simulink model "testgood"  (R2017b)
settings: Solver=VariableStepAuto  StartTime=0.0  StopTime=inf  RelTol=1e-3
libraries: dspnetwork x1, etargetslib x1
settings Model: Creator=E6320  LastModifiedBy=E6320
settings DataIOCC: SaveOutput=off  SignalLogging=off  DSMLogging=off  SaveTime=off
settings CodeAppCC: StateflowObjectComments=on

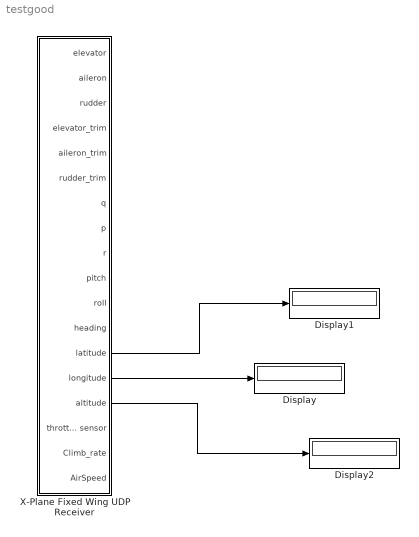
== system testgood ==
  Display : Display
  Display1 : Display
  Display2 : Display
  X-Plane Fixed Wing UDP Receiver : Subsystem  AncestorBlock=X_Plane_Communication_Library/Fixed Wing/X-Plane Fixed Wing UDP Receiver  mask{ip_adress='127.0.0.1', port_number=49004}
      mask prompts: ip_adress "Local IP Adress (default: '127.0.0.1' )"; port_number "Output Port Number (defaut: '49004')"
      mask help: This block is configured to receiver data from a fixed wing aircraft on X-Plane Flight Simulator.
      mask Help: Contact adrianobittar@gmail.com
  wires:
  X-Plane Fixed Wing UDP Receiver/14(longitude) -> Display/1
  X-Plane Fixed Wing UDP Receiver/13(latitude) -> Display1/1
  X-Plane Fixed Wing UDP Receiver/15(altitude) -> Display2/1

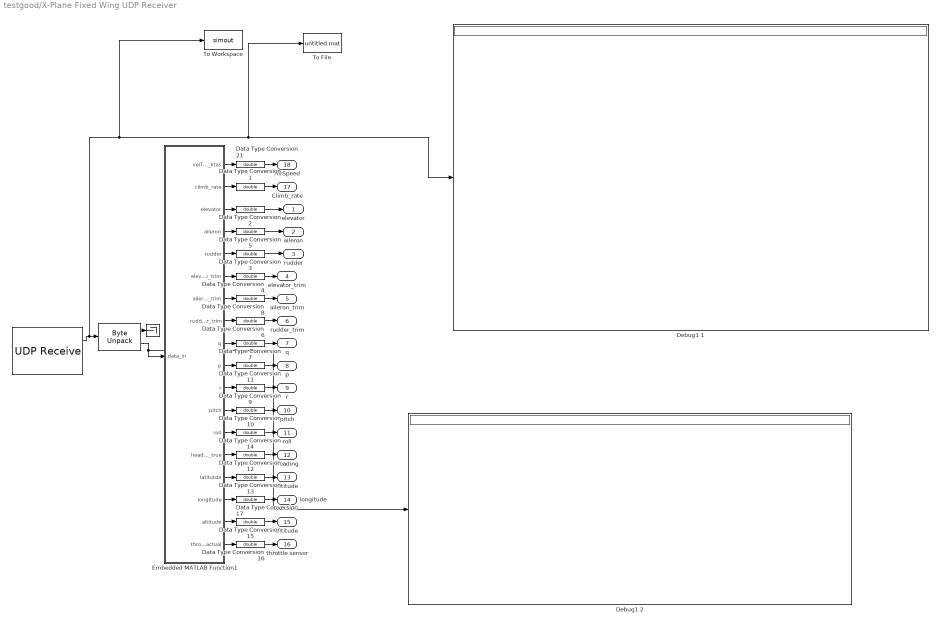
== system testgood/X-Plane Fixed Wing UDP Receiver ==
  " " : Terminator
  "    " : dspnetwork/UDP Receive  localURL='0.0.0.0'  localPort=port_number  remoteURL=ip_adress  remotePort=-1  recvBufferSize=8192  dims=293  signalDatatype=uint8  isVarSize=off  showBlockingTime=on  blockingTime=20  sampletime=0.02  blockPlatform=WINDOWS
      settings: SourceProductName=DSP System Toolbox  SourceProductBaseCode=DS
  "     " : etargetslib/Byte Unpack  dimensions={5,[9,8]}  datatypes={'uint8','single'}  byteAlign=1
  Data Type Conversion{1..17,21} (18 alike) : DataTypeConversion  OutDataTypeStr=double  SaturateOnIntegerOverflow=on
  Debug1 1 : Display
  Debug1 2 : Display
  Embedded MATLAB Function1 : MATLAB Function  TreatAsAtomicUnit=on
  To File : ToFile  SaveFormat=Timeseries
  To Workspace : ToWorkspace  VariableName=simout  SaveFormat=Timeseries  SampleTime=-1
  "elevator " : Outport
  aileron : Outport  Port=2
  rudder : Outport  Port=3
  elevator_trim : Outport  Port=4
  aileron_trim : Outport  Port=5
  rudder_trim : Outport  Port=6
  q : Outport  Port=7
  p : Outport  Port=8
  r : Outport  Port=9
  pitch : Outport  Port=10
  roll : Outport  Port=11
  heading : Outport  Port=12
  latitude : Outport  Port=13
  longitude : Outport  Port=14
  altitude : Outport  Port=15
  throttle sensor : Outport  Port=16
  Climb_rate : Outport  Port=17
  AirSpeed : Outport  Port=18
  wires:
  Data Type Conversion11/1 -> p/1
  Data Type Conversion16/1 -> throttle sensor/1
  Data Type Conversion15/1 -> altitude/1
  Data Type Conversion17/1 -> longitude/1
  Data Type Conversion14/1 -> roll/1
  Data Type Conversion13/1 -> latitude/1
  Data Type Conversion12/1 -> heading/1
  Data Type Conversion7/1 -> q/1
  Data Type Conversion6/1 -> rudder_trim/1
  Data Type Conversion4/1 -> elevator_trim/1
  Data Type Conversion3/1 -> rudder/1
  Data Type Conversion8/1 -> aileron_trim/1
  Data Type Conversion5/1 -> aileron/1
  Data Type Conversion2/1 -> "elevator "/1
  Data Type Conversion1/1 -> Climb_rate/1
  Data Type Conversion21/1 -> AirSpeed/1
  Embedded MATLAB Function1/2(climb_rate) -> Data Type Conversion1/1
  Embedded MATLAB Function1/3(elevator) -> Data Type Conversion2/1
  Embedded MATLAB Function1/4(aileron) -> Data Type Conversion5/1
  Embedded MATLAB Function1/5(rudder) -> Data Type Conversion3/1
  Embedded MATLAB Function1/6(elevator_trim) -> Data Type Conversion4/1
  Embedded MATLAB Function1/7(aileron_trim) -> Data Type Conversion8/1
  Embedded MATLAB Function1/8(rudder_trim) -> Data Type Conversion6/1
  Embedded MATLAB Function1/9(q) -> Data Type Conversion7/1
  Embedded MATLAB Function1/10(p) -> Data Type Conversion11/1
  Embedded MATLAB Function1/11(r) -> Data Type Conversion9/1
  Embedded MATLAB Function1/12(pitch) -> Data Type Conversion10/1
  Embedded MATLAB Function1/13(roll) -> Data Type Conversion14/1
  Embedded MATLAB Function1/14(heading_true) -> Data Type Conversion12/1
  Embedded MATLAB Function1/15(latitutde) -> Data Type Conversion13/1
  Embedded MATLAB Function1/16(longitude) -> Data Type Conversion17/1
  Embedded MATLAB Function1/17(altitude) -> Data Type Conversion15/1
  Embedded MATLAB Function1/18(throttle_actual) -> Data Type Conversion16/1
  Embedded MATLAB Function1/1(velTrue_ktas) -> Data Type Conversion21/1
  "     "/1 -> " "/1
  Data Type Conversion10/1 -> pitch/1
  "    "/1 -> To Workspace/1, To File/1, Debug1 1/1, "     "/1
  Data Type Conversion9/1 -> r/1
  "     "/2 -> Debug1 2/1, Embedded MATLAB Function1/1(data_in)

== matlab function testgood/X-Plane Fixed Wing UDP Receiver/Embedded MATLAB Function1 ==
  data: velTrue_ktas output; climb_rate output; data_in input; elevator output; aileron output; rudder output; elevator_trim output; aileron_trim output; rudder_trim output; q output; p output; r output; pitch output; roll output; heading_true output; latitutde output; longitude output; altitude output; throttle_actual output
function [velTrue_ktas, climb_rate,elevator, aileron, rudder, elevator_trim, aileron_trim, rudder_trim, q,p,r, pitch, roll, heading_true, latitutde, longitude, altitude, throttle_actual]   = fcn(data_in)
% This block supports the Embedded MATLAB subset.
% See the help menu for details. 


velTrue_ktas = data_in(4,1);

climb_rate = data_in(4,2);

elevator = data_in(2,3);
aileron = data_in(3,3);
rudder= data_in(4,3);


elevator_trim= data_in(2,4);
aileron_trim= data_in(3,4);
rudder_trim= data_in(4,4);

q= data_in(2,5);
p= data_in(3,5);
r= data_in(4,5);

pitch= data_in(2,6);
roll= data_in(3,6);
heading_true= data_in(4,6);

latitutde= data_in(2,7);
longitude= data_in(3,7);
altitude= data_in(4,7);


throttle_actual = data_in(2,8);
